simulink model "ec_fixed_packngo"  (Simulink 10.0)
settings: Solver=FixedStepDiscrete  StartTime=0.0  StopTime=10  RelTol=1e-3
libraries: dspsigops x1, dspadpt3 x1
settings Model: Creator=Kerry Schutz  LastModifiedBy=bhisma
settings DataIOCC: LimitDataPoints=on  SignalLoggingSaveFormat=ModelDataLogs
settings OptimizationCC: BlockReduction=off  DefaultParameterBehavior=Inlined  InlineInvariantSignals=on  ExpressionDepthLimit=2147483647  StateBitsets=on  DataBitsets=on  ZeroExternalMemoryAtStartup=off  ZeroInternalMemoryAtStartup=off  EfficientFloat2IntCast=on  LifeSpan=1  EfficientTunableParamExpr=on
settings DebuggingCC: AlgebraicLoopMsg=none  SaveWithParameterizedLinksMsg=none  SolverPrmCheckMsg=warning  FcnCallInpInsideContextMsg=warning  StateNameClashWarn=warning
settings HardwareCC: ProdBitPerInt=16  ProdBitPerPointer=16  ProdBitPerSizeT=16  ProdBitPerPtrDiffT=16  ProdIntDivRoundTo=Zero  ProdEndianess=LittleEndian  ProdWordSize=16  ProdHWDeviceType=Microchip->dsPIC  TargetHWDeviceType=32-bit Generic
settings SFSimCC: SimUseLocalCustomCode=on  SimParseCustomCode=off  MATLABDynamicMemAlloc=off  CustomCodeUndefinedFunction=FilterOut
settings RTWCC: Description=Real-Time Workshop Embedded Coder (no auto configuration)  SystemTargetFile=ert.tlc  GenCodeOnly=on  TemplateMakefile=ert_default_tmf  PostCodeGenCommand=packNGo(buildInfo)  RTWUseLocalCustomCode=on  CreateSILPILBlock=SIL
settings CodeAppCC: IgnoreCustomStorageClasses=off  CustomSymbolStrType=$N$R$M  InternalIdentifier=Classic  InlinedPrmAccess=Macros
settings ERTTargetCC: TargetFcnLib=ansi_tfl_tmw.mat  GenerateSampleERTMain=on  IncludeMdlTerminateFcn=off  SupportAbsoluteTime=off  PurelyIntegerCode=on  SupportNonFinite=off  SupportComplex=off  InlinedParameterPlacement=NonHierarchical  ERTCustomFileTemplate=example_file_process.tlc  ConvertIfToSwitch=off  SuppressUnreachableDefaultCases=off

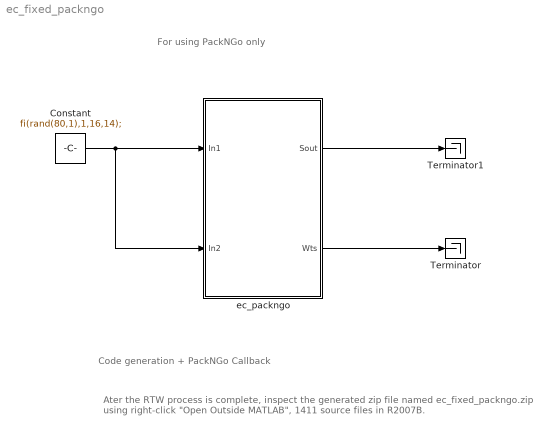
== system ec_fixed_packngo ==
  note: For using PackNGo only
  note: Code generation + PackNGo Callback
  note: Ater the RTW process is complete, inspect the generated zip file named
      | ec_fixed_packngo.zip  using right-click "Open Outside MATLAB",
      | 1411 source files in R2007B.
  Constant : Constant  Value=fi(rand(80,1),1,16,14);  VectorParams1D=off  FramePeriod=80/8000
      settings: SamplingMode=Frame based
  Terminator : Terminator
  Terminator1 : Terminator
  ec_packngo : Subsystem
  wires:
  Constant/1 -> ec_packngo/1(In1), ec_packngo/2(In2)
  ec_packngo/1(Sout) -> Terminator1/1
  ec_packngo/2(Wts) -> Terminator/1

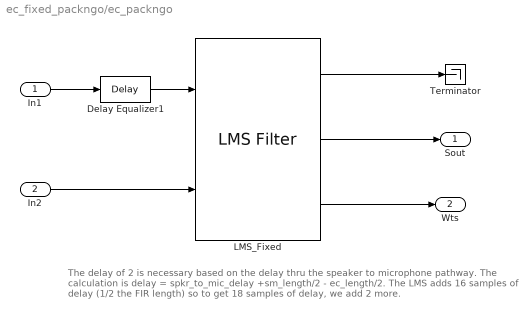
== system ec_fixed_packngo/ec_packngo ==
  note: The delay of 2 is necessary based on the delay thru the speaker to microphone pathway.
      | The calculation is delay = spkr_to_mic_delay +sm_length/2 - ec_length/2. The LMS
      | adds 16 samples of delay (1/2 the FIR length) so to get 18 samples of delay, we add 2 more.
  In1 : Inport  OutDataTypeStr=fixdt(1,16,14)
  In2 : Inport  Port=2  OutDataTypeStr=fixdt(1,16,14)
  Delay Equalizer1 : dspsigops/Delay  dly_unit=Samples  delay=2  ic_detail=off  dif_ic_for_ch=off  dif_ic_for_dly=off  ic=0  reset_popup=None
      settings: SourceProductName=DSP System Toolbox  SourceProductBaseCode=DS
  LMS_Fixed : dspadpt3/LMS Filter  Algo=LMS  L=32  stepflag=Dialog  mu=300/32768  leakage=1  ic=0  Adapt=off  resetflag=None  weights=on  secondCoeffMode=User-defined  secondCoeffWordLength=2  secondCoeffFracLength=14  accumMode=Binary point scaling  accumWordLength=16  accumFracLength=20  accum2Mode=User-defined  accum2FracLength=15  prodOutputMode=Binary point scaling  prodOutputWordLength=16  prodOutputFracLength=20  prodOutput2Mode=User-defined  prodOutput2FracLength=15  prodOutput3Mode=User-defined  prodOutput3FracLength=15  prodOutput4Mode=User-defined  prodOutput4FracLength=15  quotientMode=User-defined  quotientFracLength=20  memoryMode=Binary point scaling  memoryWordLength=16  memoryFracLength=15  roundingMode=Nearest  overflowMode=off  addnparflag=off
      settings: SourceProductName=DSP System Toolbox  SourceProductBaseCode=DS
  Terminator : Terminator
  Sout : Outport  OutDataTypeStr=fixdt(1,16,14)
  Wts : Outport  Port=2  OutDataTypeStr=fixdt(1,16,15)
  wires:
  In1/1 -> Delay Equalizer1/1
  LMS_Fixed/1 -> Terminator/1
  In2/1 -> LMS_Fixed/2
  LMS_Fixed/2 -> Sout/1
  LMS_Fixed/3 -> Wts/1
  Delay Equalizer1/1 -> LMS_Fixed/1
